simulink model "DA42HoloLensForwarder"  (R2021a)
settings: Solver=ode4  StartTime=0.0  StopTime=inf  FixedStep=0.001  RelTol=1e-3
undefined symbols (not defined in the file): Global_Sample_Time
libraries: simulink_extras x5, slrealtimeutilitieslib x2, dspnetwork x1
(part 2 of 5)

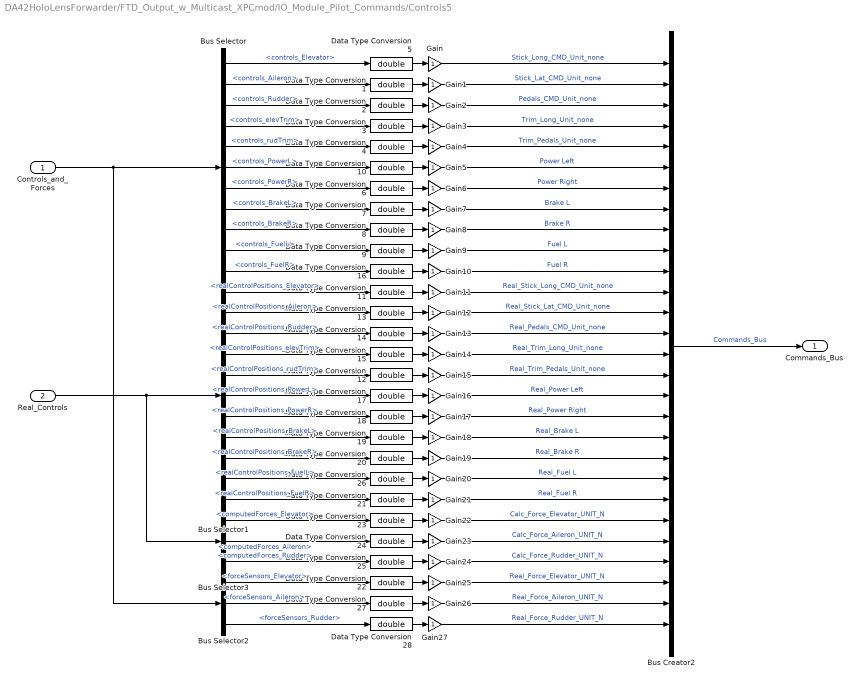
== system DA42HoloLensForwarder/FTD_Output_w_Multicast_XPCmod/IO_Module_Pilot_Commands/Controls5 ==
  Controls_and_Forces : Inport
  Real_Controls : Inport  Port=2
  Bus Creator2 : BusCreator  Inputs=28  NonVirtualBus=on
  Bus Selector : BusSelector  OutputSignals=controls_Elevator,controls_Aileron,controls_Rudder,controls_elevTrim,controls_rudTrim,controls_PowerL,controls_PowerR,controls_BrakeL,controls_BrakeR,controls_FuelL,controls_FuelR
  Bus Selector1 : BusSelector  OutputSignals=realControlPositions_Elevator,realControlPositions_Aileron,realControlPositions_Rudder,realControlPositions_elevTrim,realControlPositions_rudTrim,realControlPositions_PowerL,realControlPositions_PowerR,realControlPositions_BrakeL,realControlPositions_BrakeR,realControlPositions_FuelL,realControlPositions_FuelR
  Bus Selector2 : BusSelector  OutputSignals=forceSensors_Elevator,forceSensors_Aileron,forceSensors_Rudder
  Bus Selector3 : BusSelector  OutputSignals=computedForces_Elevator,computedForces_Aileron,computedForces_Rudder
  Data Type Conversion{1..28} (28 alike) : DataTypeConversion  OutDataTypeStr=double
  Gain{,1..27} (28 alike) : Gain
  Commands_Bus : Outport
  wires:
  Bus Selector3/3 -> Data Type Conversion25/1  "<computedForces_Rudder>"
  Bus Selector3/2 -> Data Type Conversion24/1  "<computedForces_Aileron>"
  Bus Selector3/1 -> Data Type Conversion23/1  "<computedForces_Elevator>"
  Gain10/1 -> Bus Creator2/11  "Fuel R"
  Gain9/1 -> Bus Creator2/10  "Fuel L"
  Gain8/1 -> Bus Creator2/9  "Brake R"
  Gain7/1 -> Bus Creator2/8  "Brake L"
  Gain6/1 -> Bus Creator2/7  "Power Right"
  Gain5/1 -> Bus Creator2/6  "Power Left"
  Gain4/1 -> Bus Creator2/5  "Trim_Pedals_Unit_none"
  Gain3/1 -> Bus Creator2/4  "Trim_Long_Unit_none"
  Gain2/1 -> Bus Creator2/3  "Pedals_CMD_Unit_none"
  Gain1/1 -> Bus Creator2/2  "Stick_Lat_CMD_Unit_none"
  Gain/1 -> Bus Creator2/1  "Stick_Long_CMD_Unit_none"
  Bus Creator2/1 -> Commands_Bus/1  "Commands_Bus"
  Gain11/1 -> Bus Creator2/12  "Real_Stick_Long_CMD_Unit_none"
  Gain12/1 -> Bus Creator2/13  "Real_Stick_Lat_CMD_Unit_none"
  Gain13/1 -> Bus Creator2/14  "Real_Pedals_CMD_Unit_none"
  Gain14/1 -> Bus Creator2/15  "Real_Trim_Long_Unit_none"
  Gain15/1 -> Bus Creator2/16  "Real_Trim_Pedals_Unit_none"
  Gain16/1 -> Bus Creator2/17  "Real_Power Left"
  Gain17/1 -> Bus Creator2/18  "Real_Power Right"
  Gain18/1 -> Bus Creator2/19  "Real_Brake L"
  Gain19/1 -> Bus Creator2/20  "Real_Brake R"
  Gain20/1 -> Bus Creator2/21  "Real_Fuel L"
  Gain21/1 -> Bus Creator2/22  "Real_Fuel R"
  Gain22/1 -> Bus Creator2/23  "Calc_Force_Elevator_UNIT_N"
  Gain23/1 -> Bus Creator2/24  "Calc_Force_Aileron_UNIT_N"
  Gain24/1 -> Bus Creator2/25  "Calc_Force_Rudder_UNIT_N"
  Gain25/1 -> Bus Creator2/26  "Real_Force_Elevator_UNIT_N"
  Gain26/1 -> Bus Creator2/27  "Real_Force_Aileron_UNIT_N"
  Gain27/1 -> Bus Creator2/28  "Real_Force_Rudder_UNIT_N"
  Data Type Conversion5/1 -> Gain/1
  Data Type Conversion1/1 -> Gain1/1
  Data Type Conversion2/1 -> Gain2/1
  Data Type Conversion3/1 -> Gain3/1
  Data Type Conversion4/1 -> Gain4/1
  Data Type Conversion6/1 -> Gain6/1
  Data Type Conversion7/1 -> Gain7/1
  Data Type Conversion8/1 -> Gain8/1
  Data Type Conversion9/1 -> Gain9/1
  Data Type Conversion10/1 -> Gain5/1
  Data Type Conversion16/1 -> Gain10/1
  Data Type Conversion11/1 -> Gain11/1
  Data Type Conversion13/1 -> Gain12/1
  Data Type Conversion14/1 -> Gain13/1
  Data Type Conversion15/1 -> Gain14/1
  Data Type Conversion17/1 -> Gain16/1
  Data Type Conversion18/1 -> Gain17/1
  Data Type Conversion19/1 -> Gain18/1
  Data Type Conversion20/1 -> Gain19/1
  Data Type Conversion12/1 -> Gain15/1
  Data Type Conversion26/1 -> Gain20/1
  Data Type Conversion21/1 -> Gain21/1
  Data Type Conversion23/1 -> Gain22/1
  Data Type Conversion24/1 -> Gain23/1
  Data Type Conversion25/1 -> Gain24/1
  Data Type Conversion27/1 -> Gain26/1
  Data Type Conversion28/1 -> Gain27/1
  Data Type Conversion22/1 -> Gain25/1
  Controls_and_Forces/1 -> Bus Selector/1, Bus Selector2/1
  Bus Selector/1 -> Data Type Conversion5/1  "<controls_Elevator>"
  Bus Selector/2 -> Data Type Conversion1/1  "<controls_Aileron>"
  Bus Selector/3 -> Data Type Conversion2/1  "<controls_Rudder>"
  Bus Selector/4 -> Data Type Conversion3/1  "<controls_elevTrim>"
  Bus Selector/5 -> Data Type Conversion4/1  "<controls_rudTrim>"
  Bus Selector/6 -> Data Type Conversion10/1  "<controls_PowerL>"
  Bus Selector/7 -> Data Type Conversion6/1  "<controls_PowerR>"
  Bus Selector/8 -> Data Type Conversion7/1  "<controls_BrakeL>"
  Bus Selector/9 -> Data Type Conversion8/1  "<controls_BrakeR>"
  Bus Selector/10 -> Data Type Conversion9/1  "<controls_FuelL>"
  Bus Selector/11 -> Data Type Conversion16/1  "<controls_FuelR>"
  Real_Controls/1 -> Bus Selector3/1, Bus Selector1/1
  Bus Selector1/1 -> Data Type Conversion11/1  "<realControlPositions_Elevator>"
  Bus Selector1/2 -> Data Type Conversion13/1  "<realControlPositions_Aileron>"
  Bus Selector1/3 -> Data Type Conversion14/1  "<realControlPositions_Rudder>"
  Bus Selector1/4 -> Data Type Conversion15/1  "<realControlPositions_elevTrim>"
  Bus Selector1/5 -> Data Type Conversion12/1  "<realControlPositions_rudTrim>"
  Bus Selector1/6 -> Data Type Conversion17/1  "<realControlPositions_PowerL>"
  Bus Selector1/7 -> Data Type Conversion18/1  "<realControlPositions_PowerR>"
  Bus Selector1/8 -> Data Type Conversion19/1  "<realControlPositions_BrakeL>"
  Bus Selector1/9 -> Data Type Conversion20/1  "<realControlPositions_BrakeR>"
  Bus Selector1/10 -> Data Type Conversion26/1  "<realControlPositions_FuelL>"
  Bus Selector1/11 -> Data Type Conversion21/1  "<realControlPositions_FuelR>"
  Bus Selector2/1 -> Data Type Conversion22/1  "<forceSensors_Elevator>"
  Bus Selector2/2 -> Data Type Conversion27/1  "<forceSensors_Aileron>"
  Bus Selector2/3 -> Data Type Conversion28/1  "<forceSensors_Rudder>"

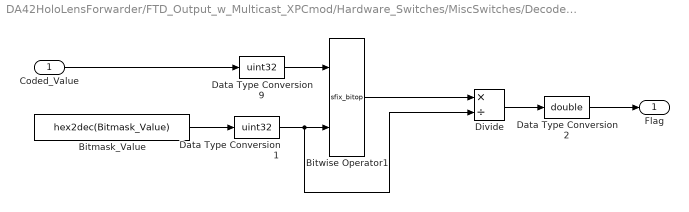
== system DA42HoloLensForwarder/FTD_Output_w_Multicast_XPCmod/Hardware_Switches/MiscSwitches/Decode_Flag ==
  Coded_Value : Inport
  Bitmask_Value : Constant  Value=hex2dec(Bitmask_Value)
  Bitwise Operator1 : S-Function  FunctionName=sfix_bitop  Parameters=UseBitMask,NumInputPorts,BitMask,BitMaskRealWorld,logicop  SFunctionDeploymentMode=off  EnableBusSupport=off  mask(Bitwise Operator){logicop=AND, UseBitMask=off, NumInputPorts=2, BitMask=bin2dec('11011001'), BitMaskRealWorld=Stored Integer}
      mask prompts: logicop "Operator:"; UseBitMask "Use bit mask ..."; NumInputPorts "Number of input ports:"; BitMask "Bit Mask"; BitMaskRealWorld "Treat mask as:"
      mask help: Perform the specified bitwise operation on the inputs. The output data type should represent zero exactly.
      mask init:
      | str = '';
      | if UseBitMask
      |   [m,n] = size(BitMask);
      |   if ischar(BitMask)
      |     len = m;
      |     n = 1;
      |   else
      |     len = m * n;
      |   end
      |   internalBitMask = zeros(m,n);
      |   if isnumeric(BitMask)
      |     for i=1:len,
      |       internalBitMask(i) = BitMask(i);
      |     end
      |   elseif ischar(BitMask)
      |     for i=1:m,
      |       internalBitMask(i) = hex2dec(BitMask(i,:));
      |     end
      |   elseif iscell(BitMask)
      |     for i=1:len,
      |       if isnumeric( BitMask{i} )
      |         internalBitMask(i) = BitMask{i};
      |       elseif ischar( BitMask{i} )
      |         internalBitMask(i) = hex2dec(BitMask{i});
      |       else
      |         errordlg(['Data type is not supported at cell item ', num2str(i) ]);
      |       end
      |     end
      |   end
      |   BitMask = internalBitMask;
      |   for i=1:len
      |     if BitMask(i) > (2^52)-1
      |       error(DAStudio.message('Simulink:blocks:BitMaskWordLengthTooLarge')); 
      |     end
      |   end 
      |   if len == 1
      |      if BitMaskRealWorld == 1 || BitMask(1) < 0
      |        str=num2str(BitMask(1));
      |      else
      |        str=['0x',dec2hex(floor(BitMask(1)))];
      |      end
      |   else
      |      str='Masks';
      |   end
      | else
      |   BitMask = 0;
      |   str='';
      | end
      mask TypeOptions logicop: AND | OR | NAND | NOR | XOR | NOT
      mask Callback logicop: fixptdialog(gcbh)
      mask Callback UseBitMask: fixptdialog(gcbh)
      mask TypeOptions BitMaskRealWorld: Real World Value | Stored Integer
      mask Display: fprintf(['Bitwise\n',logicop,'\n',str])
  Data Type Conversion1 : DataTypeConversion  OutDataTypeStr=uint32
  Data Type Conversion2 : DataTypeConversion  OutDataTypeStr=double
  Data Type Conversion9 : DataTypeConversion  OutDataTypeStr=uint32
  Divide : Product  Inputs=*/
  Flag : Outport
  wires:
  Data Type Conversion2/1 -> Flag/1
  Divide/1 -> Data Type Conversion2/1
  Data Type Conversion1/1 -> Divide/2, Bitwise Operator1/2
  Data Type Conversion9/1 -> Bitwise Operator1/1
  Bitwise Operator1/1 -> Divide/1
  Bitmask_Value/1 -> Data Type Conversion1/1
  Coded_Value/1 -> Data Type Conversion9/1

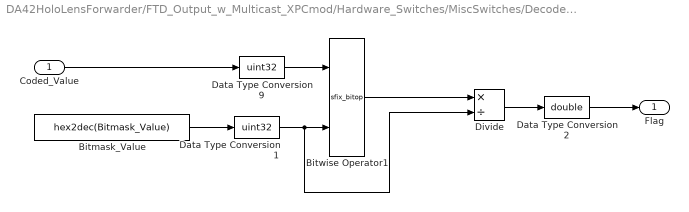
== system DA42HoloLensForwarder/FTD_Output_w_Multicast_XPCmod/Hardware_Switches/MiscSwitches/Decode_Flag1 ==
  Coded_Value : Inport
  Bitmask_Value : Constant  Value=hex2dec(Bitmask_Value)
  Bitwise Operator1 : S-Function  FunctionName=sfix_bitop  Parameters=UseBitMask,NumInputPorts,BitMask,BitMaskRealWorld,logicop  SFunctionDeploymentMode=off  EnableBusSupport=off  mask(Bitwise Operator){logicop=AND, UseBitMask=off, NumInputPorts=2, BitMask=bin2dec('11011001'), BitMaskRealWorld=Stored Integer}
      mask prompts: logicop "Operator:"; UseBitMask "Use bit mask ..."; NumInputPorts "Number of input ports:"; BitMask "Bit Mask"; BitMaskRealWorld "Treat mask as:"
      mask help: Perform the specified bitwise operation on the inputs. The output data type should represent zero exactly.
      mask init: same as DA42HoloLensForwarder/FTD_Output_w_Multicast_XPCmod/Hardware_Switches/MiscSwitches/Decode_Flag/Bitwise Operator1
      mask TypeOptions logicop: AND | OR | NAND | NOR | XOR | NOT
      mask Callback logicop: fixptdialog(gcbh)
      mask Callback UseBitMask: fixptdialog(gcbh)
      mask TypeOptions BitMaskRealWorld: Real World Value | Stored Integer
      mask Display: fprintf(['Bitwise\n',logicop,'\n',str])
  Data Type Conversion1 : DataTypeConversion  OutDataTypeStr=uint32
  Data Type Conversion2 : DataTypeConversion  OutDataTypeStr=double
  Data Type Conversion9 : DataTypeConversion  OutDataTypeStr=uint32
  Divide : Product  Inputs=*/
  Flag : Outport
  wires:
  Coded_Value/1 -> Data Type Conversion9/1
  Bitmask_Value/1 -> Data Type Conversion1/1
  Bitwise Operator1/1 -> Divide/1
  Data Type Conversion9/1 -> Bitwise Operator1/1
  Data Type Conversion1/1 -> Bitwise Operator1/2, Divide/2
  Divide/1 -> Data Type Conversion2/1
  Data Type Conversion2/1 -> Flag/1

== system DA42HoloLensForwarder/FTD_Output_w_Multicast_XPCmod/Hardware_Switches/MiscSwitches/Decode_Flag10 ==
  Coded_Value : Inport
  Bitmask_Value : Constant  Value=hex2dec(Bitmask_Value)
  Bitwise Operator1 : S-Function  FunctionName=sfix_bitop  Parameters=UseBitMask,NumInputPorts,BitMask,BitMaskRealWorld,logicop  SFunctionDeploymentMode=off  EnableBusSupport=off  mask(Bitwise Operator){logicop=AND, UseBitMask=off, NumInputPorts=2, BitMask=bin2dec('11011001'), BitMaskRealWorld=Stored Integer}
      mask prompts: logicop "Operator:"; UseBitMask "Use bit mask ..."; NumInputPorts "Number of input ports:"; BitMask "Bit Mask"; BitMaskRealWorld "Treat mask as:"
      mask help: Perform the specified bitwise operation on the inputs. The output data type should represent zero exactly.
      mask init: same as DA42HoloLensForwarder/FTD_Output_w_Multicast_XPCmod/Hardware_Switches/MiscSwitches/Decode_Flag/Bitwise Operator1
      mask TypeOptions logicop: AND | OR | NAND | NOR | XOR | NOT
      mask Callback logicop: fixptdialog(gcbh)
      mask Callback UseBitMask: fixptdialog(gcbh)
      mask TypeOptions BitMaskRealWorld: Real World Value | Stored Integer
      mask Display: fprintf(['Bitwise\n',logicop,'\n',str])
  Data Type Conversion1 : DataTypeConversion  OutDataTypeStr=uint32
  Data Type Conversion2 : DataTypeConversion  OutDataTypeStr=double
  Data Type Conversion9 : DataTypeConversion  OutDataTypeStr=uint32
  Divide : Product  Inputs=*/
  Flag : Outport
  wires:
  Coded_Value/1 -> Data Type Conversion9/1
  Bitmask_Value/1 -> Data Type Conversion1/1
  Bitwise Operator1/1 -> Divide/1
  Data Type Conversion9/1 -> Bitwise Operator1/1
  Data Type Conversion1/1 -> Bitwise Operator1/2, Divide/2
  Divide/1 -> Data Type Conversion2/1
  Data Type Conversion2/1 -> Flag/1

== system DA42HoloLensForwarder/FTD_Output_w_Multicast_XPCmod/Hardware_Switches/MiscSwitches/Decode_Flag11 ==
  Coded_Value : Inport
  Bitmask_Value : Constant  Value=hex2dec(Bitmask_Value)
  Bitwise Operator1 : S-Function  FunctionName=sfix_bitop  Parameters=UseBitMask,NumInputPorts,BitMask,BitMaskRealWorld,logicop  SFunctionDeploymentMode=off  EnableBusSupport=off  mask(Bitwise Operator){logicop=AND, UseBitMask=off, NumInputPorts=2, BitMask=bin2dec('11011001'), BitMaskRealWorld=Stored Integer}
      mask prompts: logicop "Operator:"; UseBitMask "Use bit mask ..."; NumInputPorts "Number of input ports:"; BitMask "Bit Mask"; BitMaskRealWorld "Treat mask as:"
      mask help: Perform the specified bitwise operation on the inputs. The output data type should represent zero exactly.
      mask init: same as DA42HoloLensForwarder/FTD_Output_w_Multicast_XPCmod/Hardware_Switches/MiscSwitches/Decode_Flag/Bitwise Operator1
      mask TypeOptions logicop: AND | OR | NAND | NOR | XOR | NOT
      mask Callback logicop: fixptdialog(gcbh)
      mask Callback UseBitMask: fixptdialog(gcbh)
      mask TypeOptions BitMaskRealWorld: Real World Value | Stored Integer
      mask Display: fprintf(['Bitwise\n',logicop,'\n',str])
  Data Type Conversion1 : DataTypeConversion  OutDataTypeStr=uint32
  Data Type Conversion2 : DataTypeConversion  OutDataTypeStr=double
  Data Type Conversion9 : DataTypeConversion  OutDataTypeStr=uint32
  Divide : Product  Inputs=*/
  Flag : Outport
  wires:
  Data Type Conversion2/1 -> Flag/1
  Divide/1 -> Data Type Conversion2/1
  Data Type Conversion1/1 -> Divide/2, Bitwise Operator1/2
  Data Type Conversion9/1 -> Bitwise Operator1/1
  Bitwise Operator1/1 -> Divide/1
  Bitmask_Value/1 -> Data Type Conversion1/1
  Coded_Value/1 -> Data Type Conversion9/1

== system DA42HoloLensForwarder/FTD_Output_w_Multicast_XPCmod/Hardware_Switches/MiscSwitches/Decode_Flag12 ==
  Coded_Value : Inport
  Bitmask_Value : Constant  Value=hex2dec(Bitmask_Value)
  Bitwise Operator1 : S-Function  FunctionName=sfix_bitop  Parameters=UseBitMask,NumInputPorts,BitMask,BitMaskRealWorld,logicop  SFunctionDeploymentMode=off  EnableBusSupport=off  mask(Bitwise Operator){logicop=AND, UseBitMask=off, NumInputPorts=2, BitMask=bin2dec('11011001'), BitMaskRealWorld=Stored Integer}
      mask prompts: logicop "Operator:"; UseBitMask "Use bit mask ..."; NumInputPorts "Number of input ports:"; BitMask "Bit Mask"; BitMaskRealWorld "Treat mask as:"
      mask help: Perform the specified bitwise operation on the inputs. The output data type should represent zero exactly.
      mask init: same as DA42HoloLensForwarder/FTD_Output_w_Multicast_XPCmod/Hardware_Switches/MiscSwitches/Decode_Flag/Bitwise Operator1
      mask TypeOptions logicop: AND | OR | NAND | NOR | XOR | NOT
      mask Callback logicop: fixptdialog(gcbh)
      mask Callback UseBitMask: fixptdialog(gcbh)
      mask TypeOptions BitMaskRealWorld: Real World Value | Stored Integer
      mask Display: fprintf(['Bitwise\n',logicop,'\n',str])
  Data Type Conversion1 : DataTypeConversion  OutDataTypeStr=uint32
  Data Type Conversion2 : DataTypeConversion  OutDataTypeStr=double
  Data Type Conversion9 : DataTypeConversion  OutDataTypeStr=uint32
  Divide : Product  Inputs=*/
  Flag : Outport
  wires:
  Coded_Value/1 -> Data Type Conversion9/1
  Bitmask_Value/1 -> Data Type Conversion1/1
  Bitwise Operator1/1 -> Divide/1
  Data Type Conversion9/1 -> Bitwise Operator1/1
  Data Type Conversion1/1 -> Bitwise Operator1/2, Divide/2
  Divide/1 -> Data Type Conversion2/1
  Data Type Conversion2/1 -> Flag/1

== system DA42HoloLensForwarder/FTD_Output_w_Multicast_XPCmod/Hardware_Switches/MiscSwitches/Decode_Flag13 ==
  Coded_Value : Inport
  Bitmask_Value : Constant  Value=hex2dec(Bitmask_Value)
  Bitwise Operator1 : S-Function  FunctionName=sfix_bitop  Parameters=UseBitMask,NumInputPorts,BitMask,BitMaskRealWorld,logicop  SFunctionDeploymentMode=off  EnableBusSupport=off  mask(Bitwise Operator){logicop=AND, UseBitMask=off, NumInputPorts=2, BitMask=bin2dec('11011001'), BitMaskRealWorld=Stored Integer}
      mask prompts: logicop "Operator:"; UseBitMask "Use bit mask ..."; NumInputPorts "Number of input ports:"; BitMask "Bit Mask"; BitMaskRealWorld "Treat mask as:"
      mask help: Perform the specified bitwise operation on the inputs. The output data type should represent zero exactly.
      mask init: same as DA42HoloLensForwarder/FTD_Output_w_Multicast_XPCmod/Hardware_Switches/MiscSwitches/Decode_Flag/Bitwise Operator1
      mask TypeOptions logicop: AND | OR | NAND | NOR | XOR | NOT
      mask Callback logicop: fixptdialog(gcbh)
      mask Callback UseBitMask: fixptdialog(gcbh)
      mask TypeOptions BitMaskRealWorld: Real World Value | Stored Integer
      mask Display: fprintf(['Bitwise\n',logicop,'\n',str])
  Data Type Conversion1 : DataTypeConversion  OutDataTypeStr=uint32
  Data Type Conversion2 : DataTypeConversion  OutDataTypeStr=double
  Data Type Conversion9 : DataTypeConversion  OutDataTypeStr=uint32
  Divide : Product  Inputs=*/
  Flag : Outport
  wires:
  Data Type Conversion2/1 -> Flag/1
  Divide/1 -> Data Type Conversion2/1
  Data Type Conversion1/1 -> Divide/2, Bitwise Operator1/2
  Data Type Conversion9/1 -> Bitwise Operator1/1
  Bitwise Operator1/1 -> Divide/1
  Bitmask_Value/1 -> Data Type Conversion1/1
  Coded_Value/1 -> Data Type Conversion9/1

== system DA42HoloLensForwarder/FTD_Output_w_Multicast_XPCmod/Hardware_Switches/MiscSwitches/Decode_Flag2 ==
  Coded_Value : Inport
  Bitmask_Value : Constant  Value=hex2dec(Bitmask_Value)
  Bitwise Operator1 : S-Function  FunctionName=sfix_bitop  Parameters=UseBitMask,NumInputPorts,BitMask,BitMaskRealWorld,logicop  SFunctionDeploymentMode=off  EnableBusSupport=off  mask(Bitwise Operator){logicop=AND, UseBitMask=off, NumInputPorts=2, BitMask=bin2dec('11011001'), BitMaskRealWorld=Stored Integer}
      mask prompts: logicop "Operator:"; UseBitMask "Use bit mask ..."; NumInputPorts "Number of input ports:"; BitMask "Bit Mask"; BitMaskRealWorld "Treat mask as:"
      mask help: Perform the specified bitwise operation on the inputs. The output data type should represent zero exactly.
      mask init: same as DA42HoloLensForwarder/FTD_Output_w_Multicast_XPCmod/Hardware_Switches/MiscSwitches/Decode_Flag/Bitwise Operator1
      mask TypeOptions logicop: AND | OR | NAND | NOR | XOR | NOT
      mask Callback logicop: fixptdialog(gcbh)
      mask Callback UseBitMask: fixptdialog(gcbh)
      mask TypeOptions BitMaskRealWorld: Real World Value | Stored Integer
      mask Display: fprintf(['Bitwise\n',logicop,'\n',str])
  Data Type Conversion1 : DataTypeConversion  OutDataTypeStr=uint32
  Data Type Conversion2 : DataTypeConversion  OutDataTypeStr=double
  Data Type Conversion9 : DataTypeConversion  OutDataTypeStr=uint32
  Divide : Product  Inputs=*/
  Flag : Outport
  wires:
  Coded_Value/1 -> Data Type Conversion9/1
  Bitmask_Value/1 -> Data Type Conversion1/1
  Bitwise Operator1/1 -> Divide/1
  Data Type Conversion9/1 -> Bitwise Operator1/1
  Data Type Conversion1/1 -> Bitwise Operator1/2, Divide/2
  Divide/1 -> Data Type Conversion2/1
  Data Type Conversion2/1 -> Flag/1

== system DA42HoloLensForwarder/FTD_Output_w_Multicast_XPCmod/Hardware_Switches/MiscSwitches/Decode_Flag3 ==
  Coded_Value : Inport
  Bitmask_Value : Constant  Value=hex2dec(Bitmask_Value)
  Bitwise Operator1 : S-Function  FunctionName=sfix_bitop  Parameters=UseBitMask,NumInputPorts,BitMask,BitMaskRealWorld,logicop  SFunctionDeploymentMode=off  EnableBusSupport=off  mask(Bitwise Operator){logicop=AND, UseBitMask=off, NumInputPorts=2, BitMask=bin2dec('11011001'), BitMaskRealWorld=Stored Integer}
      mask prompts: logicop "Operator:"; UseBitMask "Use bit mask ..."; NumInputPorts "Number of input ports:"; BitMask "Bit Mask"; BitMaskRealWorld "Treat mask as:"
      mask help: Perform the specified bitwise operation on the inputs. The output data type should represent zero exactly.
      mask init: same as DA42HoloLensForwarder/FTD_Output_w_Multicast_XPCmod/Hardware_Switches/MiscSwitches/Decode_Flag/Bitwise Operator1
      mask TypeOptions logicop: AND | OR | NAND | NOR | XOR | NOT
      mask Callback logicop: fixptdialog(gcbh)
      mask Callback UseBitMask: fixptdialog(gcbh)
      mask TypeOptions BitMaskRealWorld: Real World Value | Stored Integer
      mask Display: fprintf(['Bitwise\n',logicop,'\n',str])
  Data Type Conversion1 : DataTypeConversion  OutDataTypeStr=uint32
  Data Type Conversion2 : DataTypeConversion  OutDataTypeStr=double
  Data Type Conversion9 : DataTypeConversion  OutDataTypeStr=uint32
  Divide : Product  Inputs=*/
  Flag : Outport
  wires:
  Data Type Conversion2/1 -> Flag/1
  Divide/1 -> Data Type Conversion2/1
  Data Type Conversion1/1 -> Divide/2, Bitwise Operator1/2
  Data Type Conversion9/1 -> Bitwise Operator1/1
  Bitwise Operator1/1 -> Divide/1
  Bitmask_Value/1 -> Data Type Conversion1/1
  Coded_Value/1 -> Data Type Conversion9/1

== system DA42HoloLensForwarder/FTD_Output_w_Multicast_XPCmod/Hardware_Switches/MiscSwitches/Decode_Flag4 ==
  Coded_Value : Inport
  Bitmask_Value : Constant  Value=hex2dec(Bitmask_Value)
  Bitwise Operator1 : S-Function  FunctionName=sfix_bitop  Parameters=UseBitMask,NumInputPorts,BitMask,BitMaskRealWorld,logicop  SFunctionDeploymentMode=off  EnableBusSupport=off  mask(Bitwise Operator){logicop=AND, UseBitMask=off, NumInputPorts=2, BitMask=bin2dec('11011001'), BitMaskRealWorld=Stored Integer}
      mask prompts: logicop "Operator:"; UseBitMask "Use bit mask ..."; NumInputPorts "Number of input ports:"; BitMask "Bit Mask"; BitMaskRealWorld "Treat mask as:"
      mask help: Perform the specified bitwise operation on the inputs. The output data type should represent zero exactly.
      mask init: same as DA42HoloLensForwarder/FTD_Output_w_Multicast_XPCmod/Hardware_Switches/MiscSwitches/Decode_Flag/Bitwise Operator1
      mask TypeOptions logicop: AND | OR | NAND | NOR | XOR | NOT
      mask Callback logicop: fixptdialog(gcbh)
      mask Callback UseBitMask: fixptdialog(gcbh)
      mask TypeOptions BitMaskRealWorld: Real World Value | Stored Integer
      mask Display: fprintf(['Bitwise\n',logicop,'\n',str])
  Data Type Conversion1 : DataTypeConversion  OutDataTypeStr=uint32
  Data Type Conversion2 : DataTypeConversion  OutDataTypeStr=double
  Data Type Conversion9 : DataTypeConversion  OutDataTypeStr=uint32
  Divide : Product  Inputs=*/
  Flag : Outport
  wires:
  Data Type Conversion2/1 -> Flag/1
  Divide/1 -> Data Type Conversion2/1
  Data Type Conversion1/1 -> Divide/2, Bitwise Operator1/2
  Data Type Conversion9/1 -> Bitwise Operator1/1
  Bitwise Operator1/1 -> Divide/1
  Bitmask_Value/1 -> Data Type Conversion1/1
  Coded_Value/1 -> Data Type Conversion9/1

== system DA42HoloLensForwarder/FTD_Output_w_Multicast_XPCmod/Hardware_Switches/MiscSwitches/Decode_Flag5 ==
  Coded_Value : Inport
  Bitmask_Value : Constant  Value=hex2dec(Bitmask_Value)
  Bitwise Operator1 : S-Function  FunctionName=sfix_bitop  Parameters=UseBitMask,NumInputPorts,BitMask,BitMaskRealWorld,logicop  SFunctionDeploymentMode=off  EnableBusSupport=off  mask(Bitwise Operator){logicop=AND, UseBitMask=off, NumInputPorts=2, BitMask=bin2dec('11011001'), BitMaskRealWorld=Stored Integer}
      mask prompts: logicop "Operator:"; UseBitMask "Use bit mask ..."; NumInputPorts "Number of input ports:"; BitMask "Bit Mask"; BitMaskRealWorld "Treat mask as:"
      mask help: Perform the specified bitwise operation on the inputs. The output data type should represent zero exactly.
      mask init: same as DA42HoloLensForwarder/FTD_Output_w_Multicast_XPCmod/Hardware_Switches/MiscSwitches/Decode_Flag/Bitwise Operator1
      mask TypeOptions logicop: AND | OR | NAND | NOR | XOR | NOT
      mask Callback logicop: fixptdialog(gcbh)
      mask Callback UseBitMask: fixptdialog(gcbh)
      mask TypeOptions BitMaskRealWorld: Real World Value | Stored Integer
      mask Display: fprintf(['Bitwise\n',logicop,'\n',str])
  Data Type Conversion1 : DataTypeConversion  OutDataTypeStr=uint32
  Data Type Conversion2 : DataTypeConversion  OutDataTypeStr=double
  Data Type Conversion9 : DataTypeConversion  OutDataTypeStr=uint32
  Divide : Product  Inputs=*/
  Flag : Outport
  wires:
  Coded_Value/1 -> Data Type Conversion9/1
  Bitmask_Value/1 -> Data Type Conversion1/1
  Bitwise Operator1/1 -> Divide/1
  Data Type Conversion9/1 -> Bitwise Operator1/1
  Data Type Conversion1/1 -> Bitwise Operator1/2, Divide/2
  Divide/1 -> Data Type Conversion2/1
  Data Type Conversion2/1 -> Flag/1

== system DA42HoloLensForwarder/FTD_Output_w_Multicast_XPCmod/Hardware_Switches/MiscSwitches/Decode_Flag6 ==
  Coded_Value : Inport
  Bitmask_Value : Constant  Value=hex2dec(Bitmask_Value)
  Bitwise Operator1 : S-Function  FunctionName=sfix_bitop  Parameters=UseBitMask,NumInputPorts,BitMask,BitMaskRealWorld,logicop  SFunctionDeploymentMode=off  EnableBusSupport=off  mask(Bitwise Operator){logicop=AND, UseBitMask=off, NumInputPorts=2, BitMask=bin2dec('11011001'), BitMaskRealWorld=Stored Integer}
      mask prompts: logicop "Operator:"; UseBitMask "Use bit mask ..."; NumInputPorts "Number of input ports:"; BitMask "Bit Mask"; BitMaskRealWorld "Treat mask as:"
      mask help: Perform the specified bitwise operation on the inputs. The output data type should represent zero exactly.
      mask init: same as DA42HoloLensForwarder/FTD_Output_w_Multicast_XPCmod/Hardware_Switches/MiscSwitches/Decode_Flag/Bitwise Operator1
      mask TypeOptions logicop: AND | OR | NAND | NOR | XOR | NOT
      mask Callback logicop: fixptdialog(gcbh)
      mask Callback UseBitMask: fixptdialog(gcbh)
      mask TypeOptions BitMaskRealWorld: Real World Value | Stored Integer
      mask Display: fprintf(['Bitwise\n',logicop,'\n',str])
  Data Type Conversion1 : DataTypeConversion  OutDataTypeStr=uint32
  Data Type Conversion2 : DataTypeConversion  OutDataTypeStr=double
  Data Type Conversion9 : DataTypeConversion  OutDataTypeStr=uint32
  Divide : Product  Inputs=*/
  Flag : Outport
  wires:
  Coded_Value/1 -> Data Type Conversion9/1
  Bitmask_Value/1 -> Data Type Conversion1/1
  Bitwise Operator1/1 -> Divide/1
  Data Type Conversion9/1 -> Bitwise Operator1/1
  Data Type Conversion1/1 -> Bitwise Operator1/2, Divide/2
  Divide/1 -> Data Type Conversion2/1
  Data Type Conversion2/1 -> Flag/1

== system DA42HoloLensForwarder/FTD_Output_w_Multicast_XPCmod/Hardware_Switches/MiscSwitches/Decode_Flag7 ==
  Coded_Value : Inport
  Bitmask_Value : Constant  Value=hex2dec(Bitmask_Value)
  Bitwise Operator1 : S-Function  FunctionName=sfix_bitop  Parameters=UseBitMask,NumInputPorts,BitMask,BitMaskRealWorld,logicop  SFunctionDeploymentMode=off  EnableBusSupport=off  mask(Bitwise Operator){logicop=AND, UseBitMask=off, NumInputPorts=2, BitMask=bin2dec('11011001'), BitMaskRealWorld=Stored Integer}
      mask prompts: logicop "Operator:"; UseBitMask "Use bit mask ..."; NumInputPorts "Number of input ports:"; BitMask "Bit Mask"; BitMaskRealWorld "Treat mask as:"
      mask help: Perform the specified bitwise operation on the inputs. The output data type should represent zero exactly.
      mask init: same as DA42HoloLensForwarder/FTD_Output_w_Multicast_XPCmod/Hardware_Switches/MiscSwitches/Decode_Flag/Bitwise Operator1
      mask TypeOptions logicop: AND | OR | NAND | NOR | XOR | NOT
      mask Callback logicop: fixptdialog(gcbh)
      mask Callback UseBitMask: fixptdialog(gcbh)
      mask TypeOptions BitMaskRealWorld: Real World Value | Stored Integer
      mask Display: fprintf(['Bitwise\n',logicop,'\n',str])
  Data Type Conversion1 : DataTypeConversion  OutDataTypeStr=uint32
  Data Type Conversion2 : DataTypeConversion  OutDataTypeStr=double
  Data Type Conversion9 : DataTypeConversion  OutDataTypeStr=uint32
  Divide : Product  Inputs=*/
  Flag : Outport
  wires:
  Data Type Conversion2/1 -> Flag/1
  Divide/1 -> Data Type Conversion2/1
  Data Type Conversion1/1 -> Divide/2, Bitwise Operator1/2
  Data Type Conversion9/1 -> Bitwise Operator1/1
  Bitwise Operator1/1 -> Divide/1
  Bitmask_Value/1 -> Data Type Conversion1/1
  Coded_Value/1 -> Data Type Conversion9/1

== system DA42HoloLensForwarder/FTD_Output_w_Multicast_XPCmod/Hardware_Switches/MiscSwitches/Decode_Flag8 ==
  Coded_Value : Inport
  Bitmask_Value : Constant  Value=hex2dec(Bitmask_Value)
  Bitwise Operator1 : S-Function  FunctionName=sfix_bitop  Parameters=UseBitMask,NumInputPorts,BitMask,BitMaskRealWorld,logicop  SFunctionDeploymentMode=off  EnableBusSupport=off  mask(Bitwise Operator){logicop=AND, UseBitMask=off, NumInputPorts=2, BitMask=bin2dec('11011001'), BitMaskRealWorld=Stored Integer}
      mask prompts: logicop "Operator:"; UseBitMask "Use bit mask ..."; NumInputPorts "Number of input ports:"; BitMask "Bit Mask"; BitMaskRealWorld "Treat mask as:"
      mask help: Perform the specified bitwise operation on the inputs. The output data type should represent zero exactly.
      mask init: same as DA42HoloLensForwarder/FTD_Output_w_Multicast_XPCmod/Hardware_Switches/MiscSwitches/Decode_Flag/Bitwise Operator1
      mask TypeOptions logicop: AND | OR | NAND | NOR | XOR | NOT
      mask Callback logicop: fixptdialog(gcbh)
      mask Callback UseBitMask: fixptdialog(gcbh)
      mask TypeOptions BitMaskRealWorld: Real World Value | Stored Integer
      mask Display: fprintf(['Bitwise\n',logicop,'\n',str])
  Data Type Conversion1 : DataTypeConversion  OutDataTypeStr=uint32
  Data Type Conversion2 : DataTypeConversion  OutDataTypeStr=double
  Data Type Conversion9 : DataTypeConversion  OutDataTypeStr=uint32
  Divide : Product  Inputs=*/
  Flag : Outport
  wires:
  Data Type Conversion2/1 -> Flag/1
  Divide/1 -> Data Type Conversion2/1
  Data Type Conversion1/1 -> Divide/2, Bitwise Operator1/2
  Data Type Conversion9/1 -> Bitwise Operator1/1
  Bitwise Operator1/1 -> Divide/1
  Bitmask_Value/1 -> Data Type Conversion1/1
  Coded_Value/1 -> Data Type Conversion9/1

== system DA42HoloLensForwarder/FTD_Output_w_Multicast_XPCmod/Hardware_Switches/MiscSwitches/Decode_Flag9 ==
  Coded_Value : Inport
  Bitmask_Value : Constant  Value=hex2dec(Bitmask_Value)
  Bitwise Operator1 : S-Function  FunctionName=sfix_bitop  Parameters=UseBitMask,NumInputPorts,BitMask,BitMaskRealWorld,logicop  SFunctionDeploymentMode=off  EnableBusSupport=off  mask(Bitwise Operator){logicop=AND, UseBitMask=off, NumInputPorts=2, BitMask=bin2dec('11011001'), BitMaskRealWorld=Stored Integer}
      mask prompts: logicop "Operator:"; UseBitMask "Use bit mask ..."; NumInputPorts "Number of input ports:"; BitMask "Bit Mask"; BitMaskRealWorld "Treat mask as:"
      mask help: Perform the specified bitwise operation on the inputs. The output data type should represent zero exactly.
      mask init: same as DA42HoloLensForwarder/FTD_Output_w_Multicast_XPCmod/Hardware_Switches/MiscSwitches/Decode_Flag/Bitwise Operator1
      mask TypeOptions logicop: AND | OR | NAND | NOR | XOR | NOT
      mask Callback logicop: fixptdialog(gcbh)
      mask Callback UseBitMask: fixptdialog(gcbh)
      mask TypeOptions BitMaskRealWorld: Real World Value | Stored Integer
      mask Display: fprintf(['Bitwise\n',logicop,'\n',str])
  Data Type Conversion1 : DataTypeConversion  OutDataTypeStr=uint32
  Data Type Conversion2 : DataTypeConversion  OutDataTypeStr=double
  Data Type Conversion9 : DataTypeConversion  OutDataTypeStr=uint32
  Divide : Product  Inputs=*/
  Flag : Outport
  wires:
  Coded_Value/1 -> Data Type Conversion9/1
  Bitmask_Value/1 -> Data Type Conversion1/1
  Bitwise Operator1/1 -> Divide/1
  Data Type Conversion9/1 -> Bitwise Operator1/1
  Data Type Conversion1/1 -> Bitwise Operator1/2, Divide/2
  Divide/1 -> Data Type Conversion2/1
  Data Type Conversion2/1 -> Flag/1

== system DA42HoloLensForwarder/FTD_Output_w_Multicast_XPCmod/Hardware_Switches/PanelAndLegroomSwitches/Decode_Flag ==
  Coded_Value : Inport
  Bitmask_Value : Constant  Value=hex2dec(Bitmask_Value)
  Bitwise Operator1 : S-Function  FunctionName=sfix_bitop  Parameters=UseBitMask,NumInputPorts,BitMask,BitMaskRealWorld,logicop  SFunctionDeploymentMode=off  EnableBusSupport=off  mask(Bitwise Operator){logicop=AND, UseBitMask=off, NumInputPorts=2, BitMask=bin2dec('11011001'), BitMaskRealWorld=Stored Integer}
      mask prompts: logicop "Operator:"; UseBitMask "Use bit mask ..."; NumInputPorts "Number of input ports:"; BitMask "Bit Mask"; BitMaskRealWorld "Treat mask as:"
      mask help: Perform the specified bitwise operation on the inputs. The output data type should represent zero exactly.
      mask init: same as DA42HoloLensForwarder/FTD_Output_w_Multicast_XPCmod/Hardware_Switches/MiscSwitches/Decode_Flag/Bitwise Operator1
      mask TypeOptions logicop: AND | OR | NAND | NOR | XOR | NOT
      mask Callback logicop: fixptdialog(gcbh)
      mask Callback UseBitMask: fixptdialog(gcbh)
      mask TypeOptions BitMaskRealWorld: Real World Value | Stored Integer
      mask Display: fprintf(['Bitwise\n',logicop,'\n',str])
  Data Type Conversion1 : DataTypeConversion  OutDataTypeStr=uint32
  Data Type Conversion2 : DataTypeConversion  OutDataTypeStr=double
  Data Type Conversion9 : DataTypeConversion  OutDataTypeStr=uint32
  Divide : Product  Inputs=*/
  Flag : Outport
  wires:
  Coded_Value/1 -> Data Type Conversion9/1
  Bitmask_Value/1 -> Data Type Conversion1/1
  Bitwise Operator1/1 -> Divide/1
  Data Type Conversion9/1 -> Bitwise Operator1/1
  Data Type Conversion1/1 -> Bitwise Operator1/2, Divide/2
  Divide/1 -> Data Type Conversion2/1
  Data Type Conversion2/1 -> Flag/1
